simulink model "audioCancel"  (R2021b)
settings: Solver=VariableStepAuto  StartTime=0.0  StopTime=19.5  RelTol=1e-3
settings Model: Creator=IT  LastModifiedBy=82102
settings SolverCC: AlgebraicLoopSolver=TrustRegion
settings DataIOCC: ReturnWorkspaceOutputs=off
settings DebuggingCC: SFMachineParentedDataDiag=warning  ArithmeticOperatorsInVariantConditions=warning
settings SFSimCC: SimUseLocalCustomCode=off  CustomCodeUndefinedFunction=UseInterfaceOnly
settings RTWCC: RTWUseLocalCustomCode=off
settings CodeAppCC: StateflowObjectComments=on

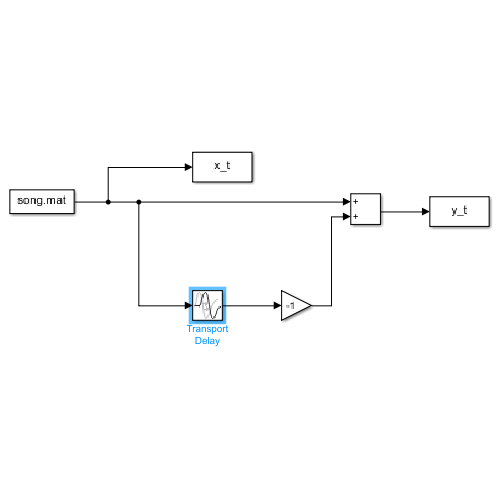
[thumbnail: Simulink's stored preview of the top-level diagram]
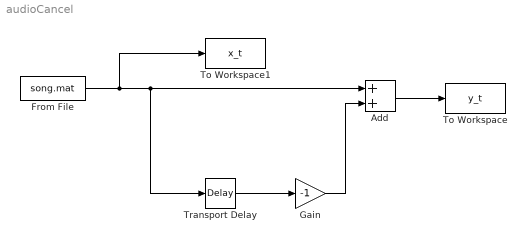
== system audioCancel ==
  Add : Sum
  From File : FromFile  FileName=song.mat  SampleTime=1/11025
  Gain : Gain  Gain=-1
  To Workspace : ToWorkspace  VariableName=y_t  SampleTime=-1
  To Workspace1 : ToWorkspace  VariableName=x_t  SampleTime=-1
  Transport Delay : TransportDelay  DelayTime=1/174.6
  wires:
  Transport Delay/1 -> Gain/1
  Gain/1 -> Add/2
  Add/1 -> To Workspace/1
  From File/1 -> Add/1, Transport Delay/1, To Workspace1/1
